simulink library "gmp_fp_utilities"  (R2024b)
settings: Solver=VariableStepAuto  StartTime=0.0  StopTime=10.0  RelTol=1e-3
undefined symbols (not defined in the file or in its folder): CMP_MAX, Deadband_Lower, Deadband_Upper, fswitch, phase_shift
libraries: simulink x2, spsCurrentMeasurementLib x1, spsVoltageMeasurementLib x1
settings Model: Creator=Javnson  LastModifiedBy=zdfxy
settings OptimizationCC: ReuseModelBlockBuffer=off
settings RTWCC: GPUComputeCapability=3.5

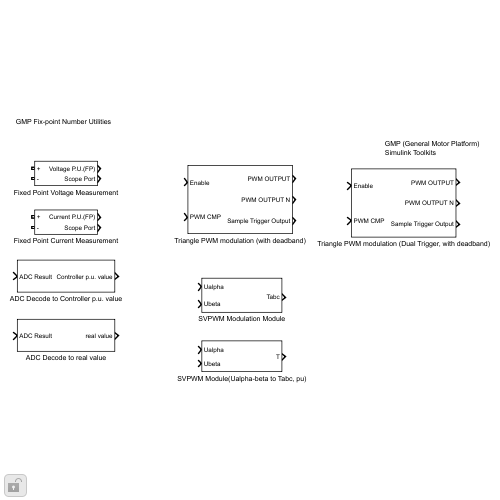
[thumbnail: Simulink's stored preview of the top-level diagram]
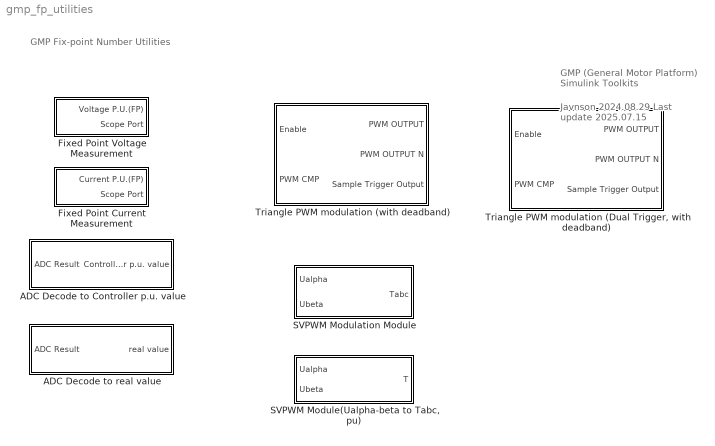
== system gmp_fp_utilities ==
  note: GMP Fix-point Number Utilities
  note: GMP (General Motor Platform)
      | Simulink Toolkits
  note: Javnson
      | 2024.08.29
      | Last update
      | 2025.07.15
  ADC Decode to Controller p.u. value : Subsystem  mask{ADC_GAIN=1, ADC_BIT=16, ADC_REF=750, ADC_BIAS=0.5}
      settings: CopyFcn=set_param(gcbh,'LinkStatus','none');
      mask DialogControl DescGroupVar Prompt: ADC Decoder
      mask DialogControl DescTextVar Prompt: GMP CTL Simulink Utilities: virtual peripherals
      mask DialogControl Control2 Prompt: Transfer adc sample result to controller p.u. value. out = gain * (adc(p.u.) - bias(p.u.)). These parameters are equal to GMP code ADC peripheral interface.
      mask DialogControl ParameterGroupVar Prompt: 参数
      mask DialogControl Control3 Prompt: ADC Voltage Gain (Scale Factor):
      mask DialogControl Control4 Prompt: ADC resolution:
      mask DialogControl Control5 Prompt: ADC reference Voltage (V), when ADC_GAIN=1, ADC_REF = ADC full scale
      mask DialogControl Control6 Prompt: ADC Bias Voltage(p.u.)
  ADC Decode to real value : Subsystem  mask{ADC_GAIN=1, ADC_BIT=16, ADC_REF=750, ADC_BIAS=0.5}
      settings: CopyFcn=set_param(gcbh,'LinkStatus','none');
      mask DialogControl DescGroupVar Prompt: ADC Decoder
      mask DialogControl DescTextVar Prompt: GMP CTL Simulink Utilities: virtual peripherals
      mask DialogControl Control2 Prompt: Transfer adc sample result to real value.
      mask DialogControl ParameterGroupVar Prompt: 参数
      mask DialogControl Control3 Prompt: ADC Voltage Gain (Scale Factor):
      mask DialogControl Control4 Prompt: ADC resolution:
      mask DialogControl Control5 Prompt: ADC reference Voltage (V), when ADC_GAIN=1, ADC_REF = ADC full scale
      mask DialogControl Control6 Prompt: ADC Bias(p.u.)
  Fixed Point Current Measurement : Subsystem  mask{PerUnit_Base=60, Q_VALUE=24}
      mask prompts: PerUnit_Base "PerUnit_Base (A) :"; Q_VALUE "Q_num"
      settings: CopyFcn=set_param(gcbh,'LinkStatus','none');
      mask DialogControl DescGroupVar Prompt: Fixed Point Voltage Measurement
      mask DialogControl DescTextVar Prompt: Measure a voltage value and transfer the real value (double type) to perunit value(int32_t).
      mask DialogControl Control2 Prompt: Parameter per unit base value:
      mask DialogControl Control3 Prompt: Fixed-point Number Q value:
  Fixed Point Voltage Measurement : Subsystem  mask{PerUnit_Base=60, Q_VALUE=24}
      mask prompts: PerUnit_Base "PerUnit_Base (V) :"; Q_VALUE "Q_num"
      mask DialogControl DescGroupVar Prompt: Fixed Point Voltage Measurement
      mask DialogControl DescTextVar Prompt: Measure a voltage value and transfer the real value (double type) to perunit value(int32_t).
      mask DialogControl Control2 Prompt: Parameter per unit base value:
      mask DialogControl Control3 Prompt: Fixed-point Number Q value:
  SVPWM Modulation Module : Subsystem  mask{half_cmp=10000}
      mask DialogControl DescGroupVar Prompt: SVPWM Modulation
      mask DialogControl DescTextVar Prompt: This Module Provide a dual level svpwm modulation tools.
      mask DialogControl Control4 Prompt: GMP CTL Simulink Utilities: virtual peripherals
      mask DialogControl Control3 Prompt: EPWM module Half Compare
  "SVPWM Module(Ualpha-beta to Tabc, pu)" : Subsystem  mask{half_cycle=10000}
      mask prompts: half_cycle "Half cycle"
      mask DialogControl DescGroupVar Prompt: SVPWM to Tabc
      mask DialogControl DescTextVar Prompt: GMP CTL Simulink Utilities: virtual peripherals
      mask DialogControl Control2 Prompt: SVPWM modulation module. Output is the compare register value.
      mask DialogControl ParameterGroupVar Prompt: Parameters:
      mask DialogControl Control3 Prompt: SVPWM Modulation Half cycle:
  "Triangle PWM modulation (Dual Trigger, with deadband)" : Subsystem  mask{fswitch=fswitch, CMP_MAX=CMP_MAX, Deadband_Upper=Deadband_Upper, Deadband_Lower=Deadband_Lower, Deadband_us=[], phase_shift=phase_shift}
      mask prompts: Deadband_us "Deadband Time: (μs)"
      mask init:
      | calculate_deadband(gcb, 'Deadband_Upper', 'Deadband_Lower',	'CMP_MAX', 'fswitch', 'Deadband_us');
      mask Callback fswitch: calculate_deadband(gcb, 'Deadband_Upper', 'Deadband_Lower',	'CMP_MAX', 'fswitch', 'Deadband_us');
      mask Callback CMP_MAX: calculate_deadband(gcb, 'Deadband_Upper', 'Deadband_Lower',	'CMP_MAX', 'fswitch', 'Deadband_us');
      mask Callback Deadband_Upper:
      | calculate_deadband(gcb, 'Deadband_Upper', 'Deadband_Lower',	'CMP_MAX', 'fswitch', 'Deadband_us');
      | 
      | % Get handle of Mask
      | %mask_obj = Simulink.Mask.get(gcb);
      | %Parameters = Simulink.Mask.get(gcb).Parameters;
      | 
      | % Get source data
      | %dead_band_up = str2double(Parameters(strcmp(get_param(gcb,'MaskNames'),'Deadband_Upper')==1).Value);
      | %dead_band_dn = str2double(Parameters(strcmp(get_param(gcb,'MaskNames'),'Deadband_Lower')==1).Value);
      | %cmp_max = str2double(Parameters(strcmp(get_param(gcb,'MaskNames'),'CMP_MAX')==1).Value);
      | %switch_freq = str2double(Parameters(strcmp(get_param(gcb,'MaskNames'),'fswitch')==1).Value);
      | 
      | % calculate deadband
      | %dead_band_us = 1/switch_freq * (dead_band_up + dead_band_dn) / cmp_max*1e6;
      | 
      | % Set result
      | %Parameters(strcmp(get_param(gcb,'MaskNames'),'Deadband_upper_us')==1).Value=num2str(dead_band_us);
      mask Callback Deadband_Lower: calculate_deadband(gcb, 'Deadband_Upper', 'Deadband_Lower',	'CMP_MAX', 'fswitch', 'Deadband_upper_us');
      mask DialogControl DescGroupVar Prompt: PWM Modulator
      mask DialogControl Control8 Prompt: GMP CTL Simulink Utilities: virtual peripherals
      mask DialogControl DescTextVar Prompt: PWM Modulator. Input PWM compare register value, output ADC trigger signal, PWM output and negtive PWM output.
      mask DialogControl ParameterGroupVar Prompt: 参数
      mask DialogControl Control2 Prompt: PWM Frequency (Hz) :
      mask DialogControl Control4 Prompt: Full Scale PWM Compare value:
      mask DialogControl Control5 Prompt: (whole period is 2 * CMP_MAX ticks)
      mask DialogControl Control3 Prompt: Deadband Range Set (CMP Value):
      mask DialogControl Control6 Prompt: Single side deadband time: DEADBAND_CMP/2/CMP_MAX/fswitch
      mask DialogControl Control7 Prompt: Initial Phase (rad)
  Triangle PWM modulation (with deadband) : Subsystem  mask{fswitch=10e3, CMP_MAX=2000, Deadband_Upper=200, Deadband_Lower=100, Deadband_us=[], phase_shift=0}
      mask prompts: Deadband_us "Deadband Time: (μs)"
      mask init:
      | calculate_deadband(gcb, 'Deadband_Upper', 'Deadband_Lower',	'CMP_MAX', 'fswitch', 'Deadband_us');
      mask Callback fswitch: calculate_deadband(gcb, 'Deadband_Upper', 'Deadband_Lower',	'CMP_MAX', 'fswitch', 'Deadband_us');
      mask Callback CMP_MAX: calculate_deadband(gcb, 'Deadband_Upper', 'Deadband_Lower',	'CMP_MAX', 'fswitch', 'Deadband_us');
      mask Callback Deadband_Upper:
      | calculate_deadband(gcb, 'Deadband_Upper', 'Deadband_Lower',	'CMP_MAX', 'fswitch', 'Deadband_us');
      | 
      | % Get handle of Mask
      | %mask_obj = Simulink.Mask.get(gcb);
      | %Parameters = Simulink.Mask.get(gcb).Parameters;
      | 
      | % Get source data
      | %dead_band_up = str2double(Parameters(strcmp(get_param(gcb,'MaskNames'),'Deadband_Upper')==1).Value);
      | %dead_band_dn = str2double(Parameters(strcmp(get_param(gcb,'MaskNames'),'Deadband_Lower')==1).Value);
      | %cmp_max = str2double(Parameters(strcmp(get_param(gcb,'MaskNames'),'CMP_MAX')==1).Value);
      | %switch_freq = str2double(Parameters(strcmp(get_param(gcb,'MaskNames'),'fswitch')==1).Value);
      | 
      | % calculate deadband
      | %dead_band_us = 1/switch_freq * (dead_band_up + dead_band_dn) / cmp_max*1e6;
      | 
      | % Set result
      | %Parameters(strcmp(get_param(gcb,'MaskNames'),'Deadband_upper_us')==1).Value=num2str(dead_band_us);
      mask Callback Deadband_Lower: calculate_deadband(gcb, 'Deadband_Upper', 'Deadband_Lower',	'CMP_MAX', 'fswitch', 'Deadband_upper_us');
      mask DialogControl DescGroupVar Prompt: PWM Modulator
      mask DialogControl Control8 Prompt: GMP CTL Simulink Utilities: virtual peripherals
      mask DialogControl DescTextVar Prompt: PWM Modulator. Input PWM compare register value, output ADC trigger signal, PWM output and negtive PWM output.
      mask DialogControl ParameterGroupVar Prompt: 参数
      mask DialogControl Control2 Prompt: PWM Frequency (Hz) :
      mask DialogControl Control4 Prompt: Full Scale PWM Compare value:
      mask DialogControl Control5 Prompt: (whole period is 2 * CMP_MAX ticks)
      mask DialogControl Control3 Prompt: Deadband Range Set (CMP Value):
      mask DialogControl Control6 Prompt: Single side deadband time: DEADBAND_CMP/2/CMP_MAX/fswitch
      mask DialogControl Control7 Prompt: Initial Phase (rad)

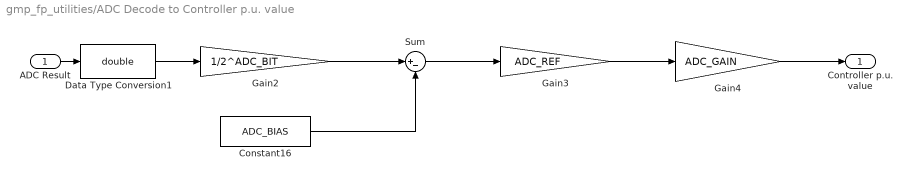
== system gmp_fp_utilities/ADC Decode to Controller p.u. value ==
  ADC Result : Inport
  Constant16 : Constant  Value=ADC_BIAS
  Data Type Conversion1 : DataTypeConversion  OutDataTypeStr=double  SaturateOnIntegerOverflow=off  RndMeth=Floor
  Gain2 : Gain  Gain=1/2^ADC_BIT
  Gain3 : Gain  Gain=ADC_REF
  Gain4 : Gain  Gain=ADC_GAIN
  Sum : Sum  Inputs=|+-
  Controller p.u. value : Outport
  wires:
  Data Type Conversion1/1 -> Gain2/1
  Gain3/1 -> Gain4/1
  Gain4/1 -> Controller p.u. value/1
  Gain2/1 -> Sum/1
  ADC Result/1 -> Data Type Conversion1/1
  Sum/1 -> Gain3/1
  Constant16/1 -> Sum/2

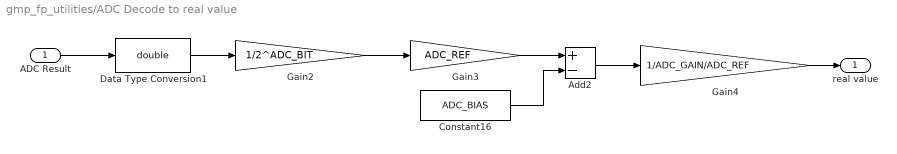
== system gmp_fp_utilities/ADC Decode to real value ==
  ADC Result : Inport
  Add2 : Sum  Inputs=+-
  Constant16 : Constant  Value=ADC_BIAS
  Data Type Conversion1 : DataTypeConversion  OutDataTypeStr=double  SaturateOnIntegerOverflow=off  RndMeth=Floor
  Gain2 : Gain  Gain=1/2^ADC_BIT
  Gain3 : Gain  Gain=ADC_REF
  Gain4 : Gain  Gain=1/ADC_GAIN/ADC_REF
  real value : Outport
  wires:
  Data Type Conversion1/1 -> Gain2/1
  Gain3/1 -> Add2/1
  Add2/1 -> Gain4/1
  Gain4/1 -> real value/1
  Constant16/1 -> Add2/2
  Gain2/1 -> Gain3/1
  ADC Result/1 -> Data Type Conversion1/1

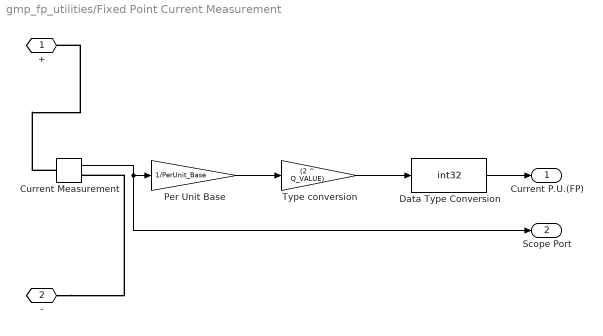
== system gmp_fp_utilities/Fixed Point Current Measurement ==
  Current Measurement : spsCurrentMeasurementLib/Current Measurement  PhasorSimulation=off  OutputType=Complex  PSBequivalent=0
  Data Type Conversion : DataTypeConversion  OutDataTypeStr=int32  ConvertRealWorld=Stored Integer (SI)  SaturateOnIntegerOverflow=off  RndMeth=Floor  LockScale=on
  Per Unit Base : Gain  Gain=1/PerUnit_Base
  Type conversion : Gain  Gain=(2 ^ Q_VALUE)
  + : PMIOPort  Side=Left
  - : PMIOPort  Port=2  Side=Left
  Current P.U.(FP) : Outport
  Scope Port : Outport  Port=2
  wires:
  Per Unit Base/1 -> Type conversion/1
  Type conversion/1 -> Data Type Conversion/1
  Data Type Conversion/1 -> Current P.U.(FP)/1
  Current Measurement/1 -> Scope Port/1, Per Unit Base/1
  connections:
  -/RConn1 -- Current Measurement/RConn1
  Current Measurement/LConn1 -- +/RConn1

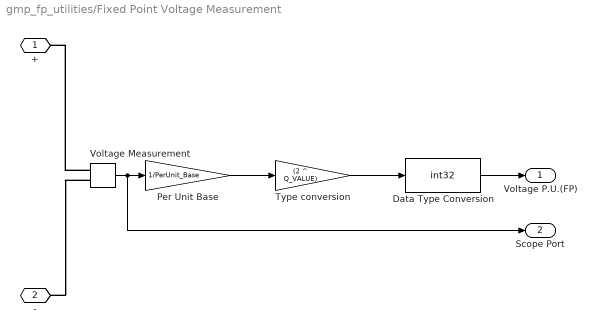
== system gmp_fp_utilities/Fixed Point Voltage Measurement ==
  Data Type Conversion : DataTypeConversion  OutDataTypeStr=int32  ConvertRealWorld=Stored Integer (SI)  SaturateOnIntegerOverflow=off  RndMeth=Floor  LockScale=on
  Per Unit Base : Gain  Gain=1/PerUnit_Base
  Type conversion : Gain  Gain=(2 ^ Q_VALUE)
  Voltage Measurement : spsVoltageMeasurementLib/Voltage Measurement  PhasorSimulation=off  OutputType=Complex  PSBequivalent=0
  + : PMIOPort  Side=Left
  - : PMIOPort  Port=2  Side=Left
  Voltage P.U.(FP) : Outport
  Scope Port : Outport  Port=2
  wires:
  Per Unit Base/1 -> Type conversion/1
  Type conversion/1 -> Data Type Conversion/1
  Data Type Conversion/1 -> Voltage P.U.(FP)/1
  Voltage Measurement/1 -> Scope Port/1, Per Unit Base/1
  connections:
  Voltage Measurement/LConn2 -- -/RConn1
  Voltage Measurement/LConn1 -- +/RConn1

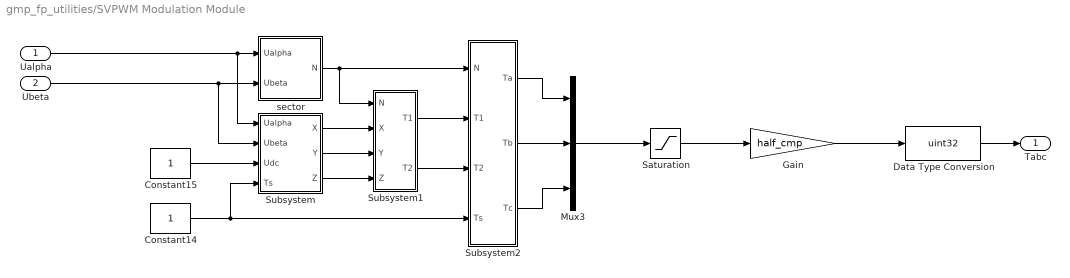
== system gmp_fp_utilities/SVPWM Modulation Module ==
  Ualpha : Inport
  Ubeta : Inport  Port=2
  Constant14 : Constant
  Constant15 : Constant
  Data Type Conversion : DataTypeConversion  OutDataTypeStr=uint32  SaturateOnIntegerOverflow=off  RndMeth=Floor
  Gain : Gain  Gain=half_cmp
  Mux3 : Mux  Inputs=3
  Saturation : Saturate  UpperLimit=1  LowerLimit=-1
  Subsystem : Subsystem
  Subsystem1 : Subsystem
  Subsystem2 : Subsystem
  sector : Subsystem
  Tabc : Outport
  wires:
  Subsystem/1(X) -> Subsystem1/2(X)
  Constant14/1 -> Subsystem2/4(Ts), Subsystem/4(Ts)
  Subsystem2/1(Ta) -> Mux3/1
  Subsystem2/3(Tc) -> Mux3/3
  Subsystem2/2(Tb) -> Mux3/2
  Ubeta/1 -> Subsystem/2(Ubeta), sector/2(Ubeta)
  sector/1(N) -> Subsystem2/1(N), Subsystem1/1(N)
  Subsystem1/1(T1) -> Subsystem2/2(T1)
  Ualpha/1 -> Subsystem/1(Ualpha), sector/1(Ualpha)
  Subsystem/2(Y) -> Subsystem1/3(Y)
  Subsystem1/2(T2) -> Subsystem2/3(T2)
  Subsystem/3(Z) -> Subsystem1/4(Z)
  Constant15/1 -> Subsystem/3(Udc)
  Mux3/1 -> Saturation/1
  Data Type Conversion/1 -> Tabc/1
  Gain/1 -> Data Type Conversion/1
  Saturation/1 -> Gain/1

== system gmp_fp_utilities/SVPWM Module(Ualpha-beta to Tabc, pu) ==
  Ualpha : Inport
  Ubeta : Inport  Port=2
  Constant : Constant  Value=half_cycle
  SVPWM Modulation : MATLAB Function  TreatAsAtomicUnit=on
  T : Outport
  wires:
  Constant/1 -> SVPWM Modulation/3(Half_cycle)
  Ualpha/1 -> SVPWM Modulation/1(Ualpha)
  Ubeta/1 -> SVPWM Modulation/2(Ubeta)
  SVPWM Modulation/1(T) -> T/1

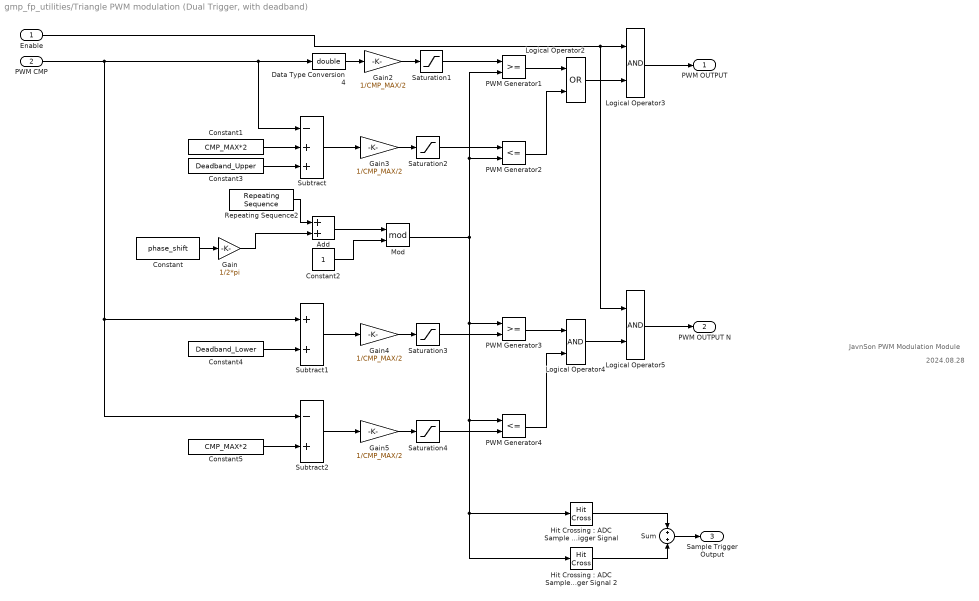
== system gmp_fp_utilities/Triangle PWM modulation (Dual Trigger, with deadband) ==
  note: 2024.08.28
  note: JavnSon PWM Modulation Module
  Enable : Inport
  PWM CMP : Inport  Port=2
  Add : Sum
  Constant : Constant  Value=phase_shift
  Constant1 : Constant  Value=CMP_MAX*2
  Constant2 : Constant
  Constant3 : Constant  Value=Deadband_Upper
  Constant4 : Constant  Value=Deadband_Lower
  Constant5 : Constant  Value=CMP_MAX*2
  Data Type Conversion4 : DataTypeConversion  OutDataTypeStr=double  SaturateOnIntegerOverflow=off  RndMeth=Floor
  Gain : Gain  Gain=1/2*pi
  Gain{2..5} (4 alike) : Gain  Gain=1/CMP_MAX/2
  Hit Crossing：ADC Sample Trigger Signal : HitCross  HitCrossingOffset=0.5  HitCrossingDirection=rising
  Hit Crossing：ADC Sample Trigger Signal 2 : HitCross  HitCrossingOffset=0.5  HitCrossingDirection=falling
  Logical Operator2 : Logic  Operator=OR  AllPortsSameDT=off  OutDataTypeStr=boolean
  Logical Operator3 : Logic  AllPortsSameDT=off  OutDataTypeStr=boolean
  Logical Operator4 : Logic  AllPortsSameDT=off  OutDataTypeStr=boolean
  Logical Operator5 : Logic  AllPortsSameDT=off  OutDataTypeStr=boolean
  Mod : Math  Operator=mod
  PWM Generator1 : RelationalOperator  OutDataTypeStr=boolean  InputSameDT=off
  PWM Generator2 : RelationalOperator  Operator=<=  OutDataTypeStr=boolean  InputSameDT=off
  PWM Generator3 : RelationalOperator  OutDataTypeStr=boolean  InputSameDT=off
  PWM Generator4 : RelationalOperator  Operator=<=  OutDataTypeStr=boolean  InputSameDT=off
  Repeating Sequence2 : simulink/Sources/Repeating Sequence  rep_seq_t=[0, 1/2/fswitch, 1/fswitch ]  rep_seq_y=[0,0.5,1]
  Saturation{1..4} (4 alike) : Saturate  UpperLimit=1  LowerLimit=0
  Subtract : Sum  Inputs=-++
  Subtract1 : Sum
  Subtract2 : Sum  Inputs=-+
  Sum : Sum  Inputs=+|+
  PWM OUTPUT : Outport
  PWM OUTPUT N : Outport  Port=2
  Sample Trigger Output : Outport  Port=3
  wires:
  PWM CMP/1 -> Subtract2/1, Subtract1/1, Subtract/1, Data Type Conversion4/1
  Data Type Conversion4/1 -> Gain2/1
  Gain2/1 -> Saturation1/1
  Saturation1/1 -> PWM Generator1/1
  PWM Generator1/1 -> Logical Operator2/1
  Logical Operator2/1 -> Logical Operator3/2
  Constant1/1 -> Subtract/2
  Constant3/1 -> Subtract/3
  PWM Generator2/1 -> Logical Operator2/2
  Gain3/1 -> Saturation2/1
  Subtract/1 -> Gain3/1
  Saturation2/1 -> PWM Generator2/1
  Constant4/1 -> Subtract1/2
  Gain4/1 -> Saturation3/1
  Subtract1/1 -> Gain4/1
  Saturation3/1 -> PWM Generator3/2
  PWM Generator3/1 -> Logical Operator4/1
  Constant5/1 -> Subtract2/2
  Saturation4/1 -> PWM Generator4/2
  Gain5/1 -> Saturation4/1
  Subtract2/1 -> Gain5/1
  PWM Generator4/1 -> Logical Operator4/2
  Logical Operator4/1 -> Logical Operator5/2
  Mod/1 -> PWM Generator2/2, PWM Generator1/2, PWM Generator3/1, Hit Crossing：ADC Sample Trigger Signal 2/1, Hit Crossing：ADC Sample Trigger Signal/1, PWM Generator4/1
  Enable/1 -> Logical Operator5/1, Logical Operator3/1
  Logical Operator5/1 -> PWM OUTPUT N/1
  Logical Operator3/1 -> PWM OUTPUT/1
  Repeating Sequence2/1 -> Add/1
  Gain/1 -> Add/2
  Add/1 -> Mod/1
  Constant2/1 -> Mod/2
  Constant/1 -> Gain/1
  Hit Crossing：ADC Sample Trigger Signal/1 -> Sum/1
  Hit Crossing：ADC Sample Trigger Signal 2/1 -> Sum/2
  Sum/1 -> Sample Trigger Output/1

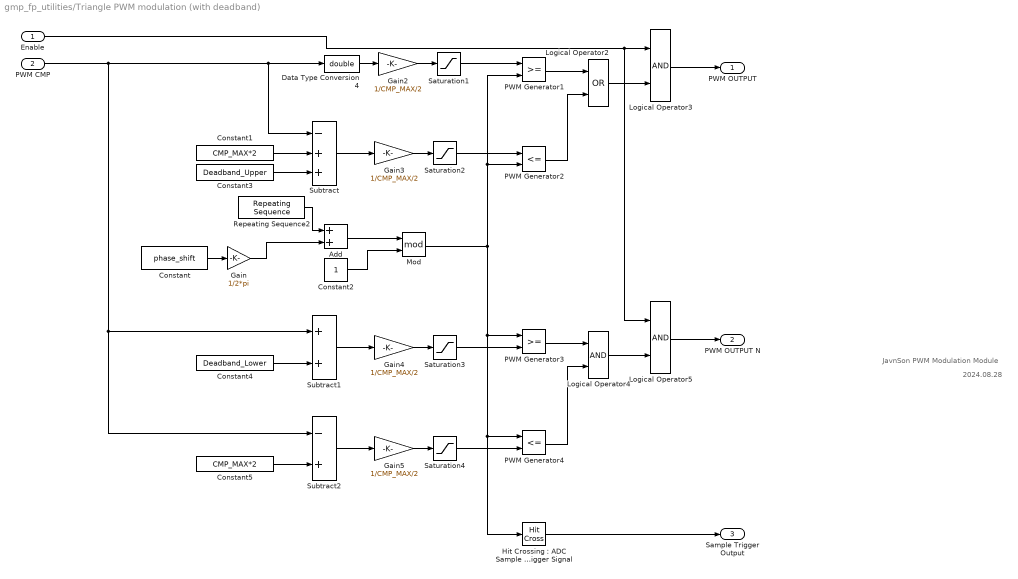
== system gmp_fp_utilities/Triangle PWM modulation (with deadband) ==
  note: 2024.08.28
  note: JavnSon PWM Modulation Module
  Enable : Inport
  PWM CMP : Inport  Port=2
  Add : Sum
  Constant : Constant  Value=phase_shift
  Constant1 : Constant  Value=CMP_MAX*2
  Constant2 : Constant
  Constant3 : Constant  Value=Deadband_Upper
  Constant4 : Constant  Value=Deadband_Lower
  Constant5 : Constant  Value=CMP_MAX*2
  Data Type Conversion4 : DataTypeConversion  OutDataTypeStr=double  SaturateOnIntegerOverflow=off  RndMeth=Floor
  Gain : Gain  Gain=1/2*pi
  Gain{2..5} (4 alike) : Gain  Gain=1/CMP_MAX/2
  Hit Crossing：ADC Sample Trigger Signal : HitCross  HitCrossingOffset=0.5  HitCrossingDirection=rising
  Logical Operator2 : Logic  Operator=OR  AllPortsSameDT=off  OutDataTypeStr=boolean
  Logical Operator3 : Logic  AllPortsSameDT=off  OutDataTypeStr=boolean
  Logical Operator4 : Logic  AllPortsSameDT=off  OutDataTypeStr=boolean
  Logical Operator5 : Logic  AllPortsSameDT=off  OutDataTypeStr=boolean
  Mod : Math  Operator=mod
  PWM Generator1 : RelationalOperator  OutDataTypeStr=boolean  InputSameDT=off
  PWM Generator2 : RelationalOperator  Operator=<=  OutDataTypeStr=boolean  InputSameDT=off
  PWM Generator3 : RelationalOperator  OutDataTypeStr=boolean  InputSameDT=off
  PWM Generator4 : RelationalOperator  Operator=<=  OutDataTypeStr=boolean  InputSameDT=off
  Repeating Sequence2 : simulink/Sources/Repeating Sequence  rep_seq_t=[0, 1/2/fswitch, 1/fswitch ]  rep_seq_y=[0,0.5,1]
  Saturation{1..4} (4 alike) : Saturate  UpperLimit=1  LowerLimit=0
  Subtract : Sum  Inputs=-++
  Subtract1 : Sum
  Subtract2 : Sum  Inputs=-+
  PWM OUTPUT : Outport
  PWM OUTPUT N : Outport  Port=2
  Sample Trigger Output : Outport  Port=3
  wires:
  PWM CMP/1 -> Subtract2/1, Subtract1/1, Subtract/1, Data Type Conversion4/1
  Data Type Conversion4/1 -> Gain2/1
  Gain2/1 -> Saturation1/1
  Saturation1/1 -> PWM Generator1/1
  PWM Generator1/1 -> Logical Operator2/1
  Logical Operator2/1 -> Logical Operator3/2
  Constant1/1 -> Subtract/2
  Constant3/1 -> Subtract/3
  PWM Generator2/1 -> Logical Operator2/2
  Gain3/1 -> Saturation2/1
  Subtract/1 -> Gain3/1
  Saturation2/1 -> PWM Generator2/1
  Constant4/1 -> Subtract1/2
  Gain4/1 -> Saturation3/1
  Subtract1/1 -> Gain4/1
  Saturation3/1 -> PWM Generator3/2
  PWM Generator3/1 -> Logical Operator4/1
  Constant5/1 -> Subtract2/2
  Saturation4/1 -> PWM Generator4/2
  Gain5/1 -> Saturation4/1
  Subtract2/1 -> Gain5/1
  PWM Generator4/1 -> Logical Operator4/2
  Logical Operator4/1 -> Logical Operator5/2
  Mod/1 -> PWM Generator2/2, PWM Generator1/2, PWM Generator3/1, Hit Crossing：ADC Sample Trigger Signal/1, PWM Generator4/1
  Enable/1 -> Logical Operator5/1, Logical Operator3/1
  Logical Operator5/1 -> PWM OUTPUT N/1
  Logical Operator3/1 -> PWM OUTPUT/1
  Hit Crossing：ADC Sample Trigger Signal/1 -> Sample Trigger Output/1
  Repeating Sequence2/1 -> Add/1
  Gain/1 -> Add/2
  Add/1 -> Mod/1
  Constant2/1 -> Mod/2
  Constant/1 -> Gain/1

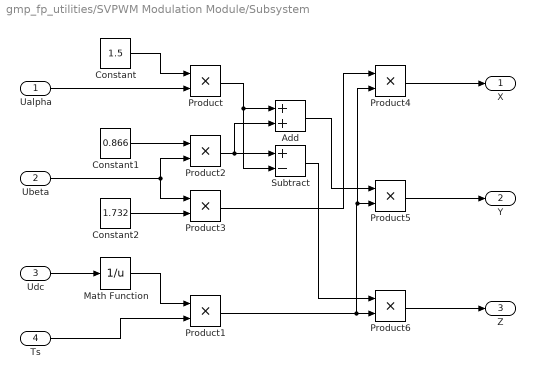
== system gmp_fp_utilities/SVPWM Modulation Module/Subsystem ==
  Ualpha : Inport
  Ubeta : Inport  Port=2
  Udc : Inport  Port=3
  Ts : Inport  Port=4
  Add : Sum
  Constant : Constant  Value=1.5
  Constant1 : Constant  Value=0.866
  Constant2 : Constant  Value=1.732
  Math Function : Math  Operator=reciprocal
  Product{,1..6} (7 alike) : Product
  Subtract : Sum  Inputs=+-
  X : Outport
  Y : Outport  Port=2
  Z : Outport  Port=3
  wires:
  Product1/1 -> Product4/2, Product5/2, Product6/2
  Ts/1 -> Product1/2
  Product6/1 -> Z/1
  Add/1 -> Product5/1
  Ualpha/1 -> Product/2
  Math Function/1 -> Product1/1
  Product2/1 -> Subtract/1, Add/2
  Product4/1 -> X/1
  Product3/1 -> Product4/1
  Constant/1 -> Product/1
  Constant1/1 -> Product2/1
  Ubeta/1 -> Product3/1, Product2/2
  Product5/1 -> Y/1
  Product/1 -> Add/1, Subtract/2
  Constant2/1 -> Product3/2
  Udc/1 -> Math Function/1
  Subtract/1 -> Product6/1

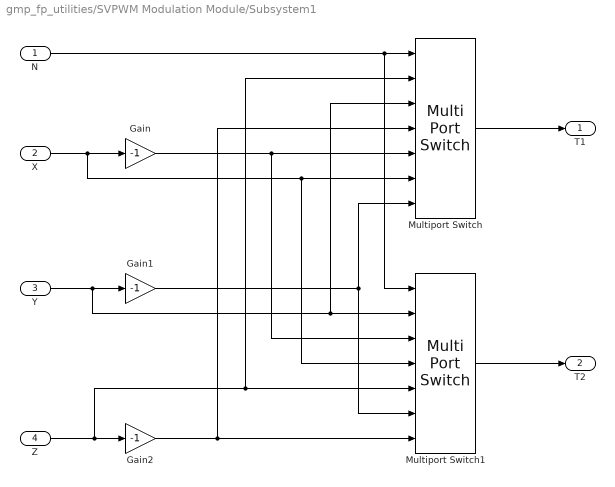
== system gmp_fp_utilities/SVPWM Modulation Module/Subsystem1 ==
  N : Inport
  X : Inport  Port=2
  Y : Inport  Port=3
  Z : Inport  Port=4
  Gain : Gain  Gain=-1
  Gain1 : Gain  Gain=-1
  Gain2 : Gain  Gain=-1
  Multiport Switch : MultiPortSwitch  Inputs=6  DiagnosticForDefault=None  SaturateOnIntegerOverflow=off  InputSameDT=off
  Multiport Switch1 : MultiPortSwitch  Inputs=6  DiagnosticForDefault=None  SaturateOnIntegerOverflow=off  InputSameDT=off
  T1 : Outport
  T2 : Outport  Port=2
  wires:
  Multiport Switch1/1 -> T2/1
  X/1 -> Multiport Switch1/4, Multiport Switch/6, Gain/1
  Y/1 -> Gain1/1, Multiport Switch/3, Multiport Switch1/2
  Z/1 -> Gain2/1, Multiport Switch/2, Multiport Switch1/5
  Gain/1 -> Multiport Switch1/3, Multiport Switch/5
  Gain2/1 -> Multiport Switch/4, Multiport Switch1/7
  N/1 -> Multiport Switch1/1, Multiport Switch/1
  Gain1/1 -> Multiport Switch1/6, Multiport Switch/7
  Multiport Switch/1 -> T1/1

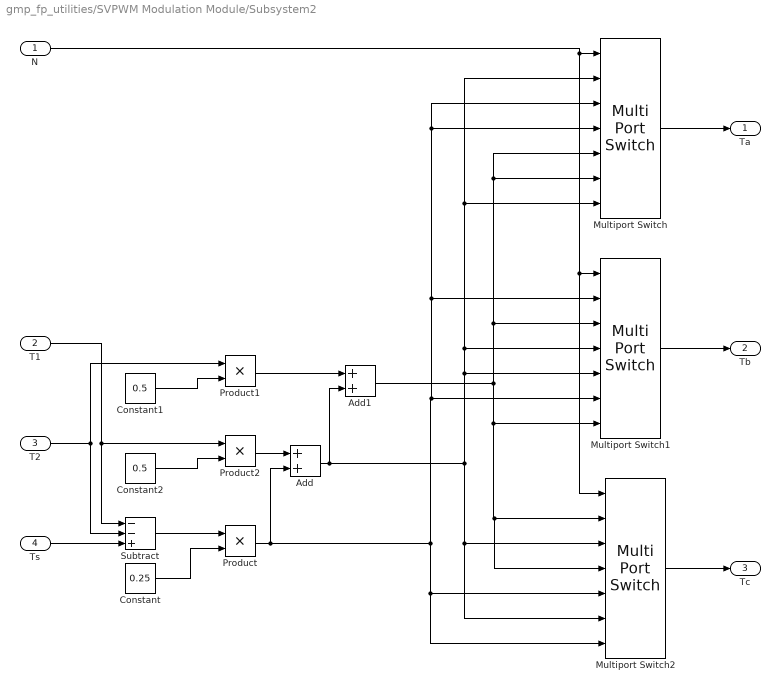
== system gmp_fp_utilities/SVPWM Modulation Module/Subsystem2 ==
  N : Inport
  T1 : Inport  Port=2  Interpolate=off
  T2 : Inport  Port=3
  Ts : Inport  Port=4
  Add : Sum
  Add1 : Sum
  Constant : Constant  Value=0.25
  Constant1 : Constant  Value=0.5
  Constant2 : Constant  Value=0.5
  Multiport Switch : MultiPortSwitch  Inputs=6  DiagnosticForDefault=None  SaturateOnIntegerOverflow=off  InputSameDT=off
  Multiport Switch1 : MultiPortSwitch  Inputs=6  DiagnosticForDefault=None  SaturateOnIntegerOverflow=off  InputSameDT=off
  Multiport Switch2 : MultiPortSwitch  Inputs=6  DiagnosticForDefault=None  SaturateOnIntegerOverflow=off  InputSameDT=off
  Product : Product
  Product1 : Product
  Product2 : Product
  Subtract : Sum  Inputs=--+
  Ta : Outport
  Tb : Outport  Port=2
  Tc : Outport  Port=3
  wires:
  Subtract/1 -> Product/1
  Product1/1 -> Add1/1
  T2/1 -> Product1/1, Subtract/2
  Product/1 -> Add/2, Multiport Switch2/5, Multiport Switch2/7, Multiport Switch/4, Multiport Switch/3, Multiport Switch1/2, Multiport Switch1/6
  Multiport Switch2/1 -> Tc/1
  Add1/1 -> Multiport Switch2/4, Multiport Switch2/2, Multiport Switch1/7, Multiport Switch1/3, Multiport Switch/6, Multiport Switch/5
  N/1 -> Multiport Switch2/1, Multiport Switch1/1, Multiport Switch/1
  Multiport Switch/1 -> Ta/1
  Constant/1 -> Product/2
  Constant2/1 -> Product2/2
  Add/1 -> Add1/2, Multiport Switch1/5, Multiport Switch/7, Multiport Switch/2, Multiport Switch1/4, Multiport Switch2/6, Multiport Switch2/3
  Multiport Switch1/1 -> Tb/1
  Product2/1 -> Add/1
  Constant1/1 -> Product1/2
  T1/1 -> Product2/1, Subtract/1
  Ts/1 -> Subtract/3

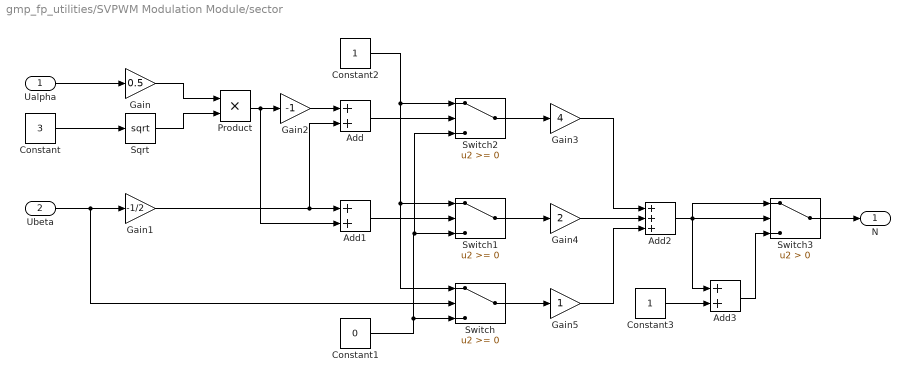
== system gmp_fp_utilities/SVPWM Modulation Module/sector ==
  Ualpha : Inport
  Ubeta : Inport  Port=2
  Add : Sum
  Add1 : Sum
  Add2 : Sum  Inputs=+++
  Add3 : Sum
  Constant : Constant  Value=3
  Constant1 : Constant  Value=0
  Constant2 : Constant
  Constant3 : Constant
  Gain : Gain  Gain=0.5
  Gain1 : Gain  Gain=-1/2
  Gain2 : Gain  Gain=-1
  Gain3 : Gain  Gain=4
  Gain4 : Gain  Gain=2
  Gain5 : Gain
  Product : Product
  Sqrt : Sqrt
  Switch : Switch  SaturateOnIntegerOverflow=off  InputSameDT=off
  Switch1 : Switch  SaturateOnIntegerOverflow=off  InputSameDT=off
  Switch2 : Switch  SaturateOnIntegerOverflow=off  InputSameDT=off
  Switch3 : Switch  Criteria=u2 > Threshold  SaturateOnIntegerOverflow=off  InputSameDT=off
  N : Outport
  wires:
  Gain1/1 -> Add1/1, Add/2
  Constant1/1 -> Switch2/3, Switch1/3, Switch/3
  Gain2/1 -> Add/1
  Gain/1 -> Product/1
  Constant3/1 -> Add3/2
  Add/1 -> Switch2/2
  Product/1 -> Add1/2, Gain2/1
  Sqrt/1 -> Product/2
  Ubeta/1 -> Switch/2, Gain1/1
  Switch/1 -> Gain5/1
  Switch2/1 -> Gain3/1
  Add3/1 -> Switch3/3
  Add2/1 -> Switch3/1, Add3/1, Switch3/2
  Switch3/1 -> N/1
  Gain3/1 -> Add2/1
  Add1/1 -> Switch1/2
  Switch1/1 -> Gain4/1
  Gain4/1 -> Add2/2
  Constant/1 -> Sqrt/1
  Gain5/1 -> Add2/3
  Constant2/1 -> Switch/1, Switch1/1, Switch2/1
  Ualpha/1 -> Gain/1

== matlab function gmp_fp_utilities/SVPWM Module(Ualpha-beta to Tabc, pu)/SVPWM Modulation ==
  data: Ualpha input; T output; Ubeta input; Half_cycle input
function T = fcn(Ualpha, Ubeta, Half_cycle)

T = zeros(3,1);

Ualpha_tmp = -Ualpha/2;
Ubeta_tmp = Ubeta*sqrt(3)/2;

Ua = Ualpha;
Ub = Ualpha_tmp + Ubeta_tmp;
Uc = Ualpha_tmp - Ubeta_tmp;


if (Ua > Ub)
    Umax = Ua;
    Umin = Ub;
else
    Umax = Ub;
    Umin = Ua;
end

if (Uc > Umax)
    Umax = Uc;
elseif (Uc < Umin)
    Umin = Uc;
end

Ucom = (Umax + Umin)/2;

T(1) = Ua - Ucom;
T(2) = Ub - Ucom;
T(3) = Uc - Ucom;

T = (T + 0.5) .* Half_cycle ;
end
